simulink model "Controller_CompareModelWithMeasurement"  (R2019b)
settings: Solver=VariableStepAuto  StartTime=0.0  StopTime=10.0  RelTol=1e-3
values from neighbouring files (symbols this model uses):
  I_init = 0    [PerformSimulation_CompareModelWithMeasurement.m]
undefined symbols (not defined in the file or in its folder): denc_mi, numc_mi, ts
settings Model: Creator=Duin home  LastModifiedBy=Duin home

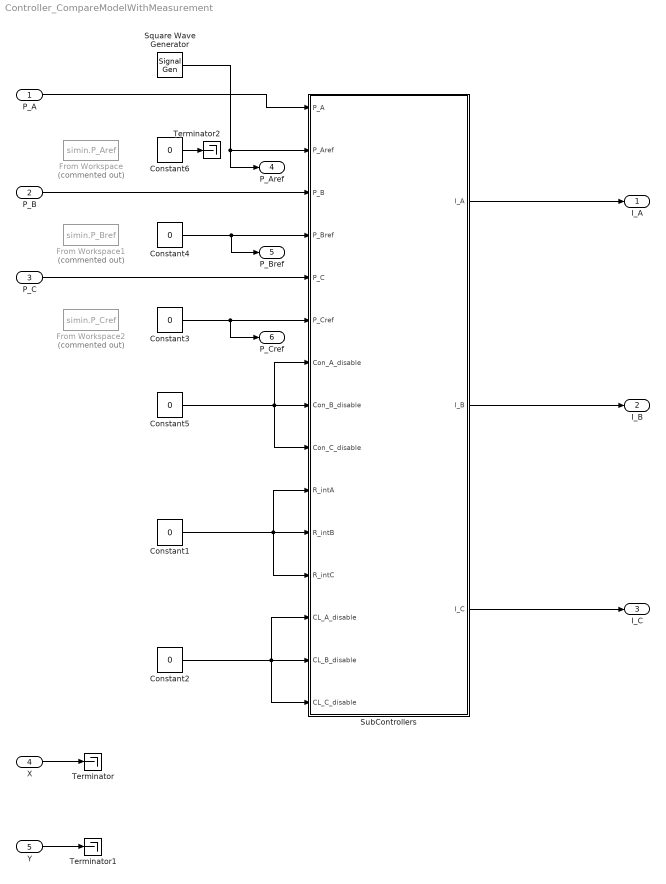
== system Controller_CompareModelWithMeasurement ==
  P_A : Inport
  P_B : Inport  Port=2
  P_C : Inport  Port=3
  X : Inport  Port=4
  Y : Inport  Port=5
  Constant{1..6} (6 alike) : Constant  Value=0
  From Workspace : FromWorkspace  Commented=on  VariableName=simin.P_Aref  SampleTime=ts  Interpolate=off  OutputAfterFinalValue=Holding final value
  From Workspace1 : FromWorkspace  Commented=on  VariableName=simin.P_Bref  SampleTime=ts  Interpolate=off  OutputAfterFinalValue=Holding final value
  From Workspace2 : FromWorkspace  Commented=on  VariableName=simin.P_Cref  SampleTime=ts  Interpolate=off  OutputAfterFinalValue=Holding final value
  Square Wave Generator : SignalGenerator  WaveForm=square  Amplitude=0.025  Frequency=0.5  Units=rad/sec
  SubControllers : Subsystem
  Terminator : Terminator
  Terminator1 : Terminator
  Terminator2 : Terminator
  I_A : Outport
  I_B : Outport  Port=2
  I_C : Outport  Port=3
  P_Aref : Outport  Port=4
  P_Bref : Outport  Port=5
  P_Cref : Outport  Port=6
  wires:
  P_B/1 -> SubControllers/3(P_B)
  Square Wave Generator/1 -> P_Aref/1, SubControllers/2(P_Aref)
  Constant4/1 -> P_Bref/1, SubControllers/4("P_Bref ")
  P_A/1 -> SubControllers/1(P_A)
  Constant5/1 -> SubControllers/7(Con_A_disable), SubControllers/9(Con_C_disable), SubControllers/8(Con_B_disable)
  Constant3/1 -> P_Cref/1, SubControllers/6(P_Cref)
  SubControllers/2(I_B) -> I_B/1
  P_C/1 -> SubControllers/5(P_C)
  Constant1/1 -> SubControllers/11(R_intB), SubControllers/10(R_intA), SubControllers/12(R_intC)
  Constant2/1 -> SubControllers/13(CL_A_disable), SubControllers/15(CL_C_disable), SubControllers/14(CL_B_disable)
  SubControllers/3(I_C) -> I_C/1
  SubControllers/1(I_A) -> I_A/1
  X/1 -> Terminator/1
  Y/1 -> Terminator1/1
  Constant6/1 -> Terminator2/1

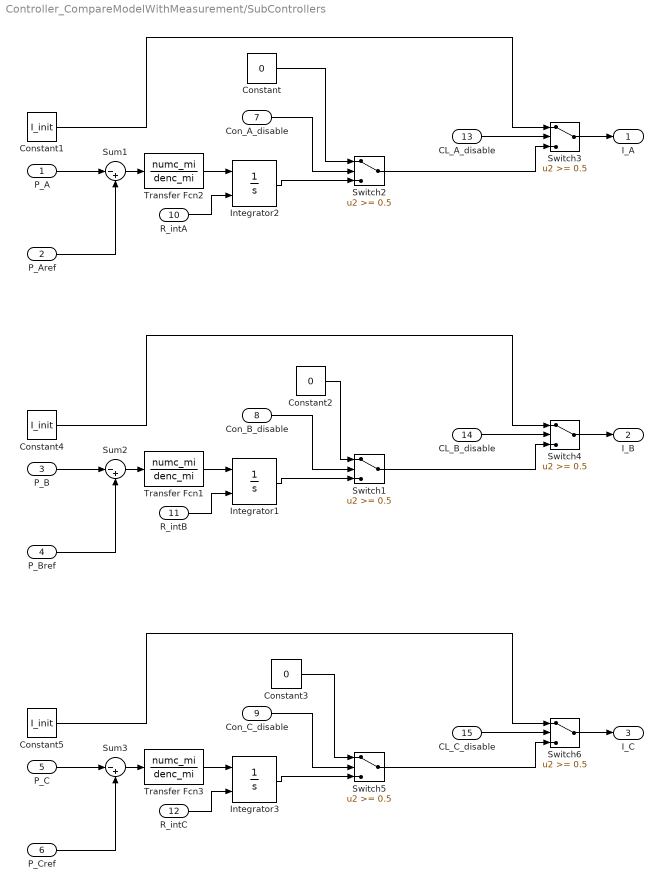
== system Controller_CompareModelWithMeasurement/SubControllers ==
  P_A : Inport
  P_Aref : Inport  Port=2
  P_B : Inport  Port=3
  "P_Bref " : Inport  Port=4
  P_C : Inport  Port=5
  P_Cref : Inport  Port=6
  Con_A_disable : Inport  Port=7
  Con_B_disable : Inport  Port=8
  Con_C_disable : Inport  Port=9
  R_intA : Inport  Port=10
  R_intB : Inport  Port=11
  R_intC : Inport  Port=12
  CL_A_disable : Inport  Port=13
  CL_B_disable : Inport  Port=14
  CL_C_disable : Inport  Port=15
  Constant : Constant  Value=0
  Constant1 : Constant  Value=I_init
  Constant2 : Constant  Value=0
  Constant3 : Constant  Value=0
  Constant4 : Constant  Value=I_init
  Constant5 : Constant  Value=I_init
  Integrator1 : Integrator  ExternalReset=rising  LimitOutput=on  UpperSaturationLimit=3  LowerSaturationLimit=-3
  Integrator2 : Integrator  ExternalReset=rising  LimitOutput=on  UpperSaturationLimit=3  LowerSaturationLimit=-3
  Integrator3 : Integrator  ExternalReset=rising  LimitOutput=on  UpperSaturationLimit=3  LowerSaturationLimit=-3
  Sum1 : Sum  Inputs=|-+  SaturateOnIntegerOverflow=on
  Sum2 : Sum  Inputs=|-+  SaturateOnIntegerOverflow=on
  Sum3 : Sum  Inputs=|-+  SaturateOnIntegerOverflow=on
  Switch{1..6} (6 alike) : Switch  Threshold=0.5
  Transfer Fcn1 : TransferFcn  Numerator=numc_mi  Denominator=denc_mi
  Transfer Fcn2 : TransferFcn  Numerator=numc_mi  Denominator=denc_mi
  Transfer Fcn3 : TransferFcn  Numerator=numc_mi  Denominator=denc_mi
  I_A : Outport
  I_B : Outport  Port=2
  I_C : Outport  Port=3
  wires:
  Switch1/1 -> Switch4/3
  R_intA/1 -> Integrator2/2
  Integrator3/1 -> Switch5/3
  Con_C_disable/1 -> Switch5/2
  Constant5/1 -> Switch6/1
  P_C/1 -> Sum3/1
  Transfer Fcn3/1 -> Integrator3/1
  Switch5/1 -> Switch6/3
  Switch6/1 -> I_C/1
  Sum3/1 -> Transfer Fcn3/1
  Integrator1/1 -> Switch1/3
  Constant1/1 -> Switch3/1
  Constant3/1 -> Switch5/1
  CL_C_disable/1 -> Switch6/2
  R_intC/1 -> Integrator3/2
  Transfer Fcn1/1 -> Integrator1/1
  Sum2/1 -> Transfer Fcn1/1
  Con_B_disable/1 -> Switch1/2
  R_intB/1 -> Integrator1/2
  P_B/1 -> Sum2/1
  Constant2/1 -> Switch1/1
  CL_A_disable/1 -> Switch3/2
  Constant4/1 -> Switch4/1
  CL_B_disable/1 -> Switch4/2
  P_A/1 -> Sum1/1
  P_Aref/1 -> Sum1/2
  Switch2/1 -> Switch3/3
  Constant/1 -> Switch2/1
  Transfer Fcn2/1 -> Integrator2/1
  Switch3/1 -> I_A/1
  Integrator2/1 -> Switch2/3
  Con_A_disable/1 -> Switch2/2
  Sum1/1 -> Transfer Fcn2/1
  P_Cref/1 -> Sum3/2
  "P_Bref "/1 -> Sum2/2
  Switch4/1 -> I_B/1
